simulink library "simeventstiming1"  (Simulink 6.6)
undefined symbols (not defined in the file or in its folder): des_support, gcbh
settings Model: Creator=mclune  LastModifiedBy=aapte  ExtModeAutoUpdateStatusClock=off

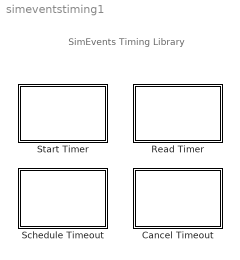
== system simeventstiming1 ==
  note: SimEvents Timing Library
  Cancel Timeout : Subsystem  Priority=0  LoadFcn=des_support('desLoadFcn',gcbh)  StartFcn=des_support('desStartFcn',gcbh)  StopFcn=des_support('desStopFcn',gcbh)  mask(Cancel Timeout){TimeoutTag=TO1, TimeoutModeOption=Continue, TimeoutCancelledOption=Error, StatNumberDeparted=Off, StatTimeoutNumberDeparted=Off, StatResidualTimeout=Off, StatAverageResidualTimeout=Off}
      mask prompts: TimeoutTag "Timeout tag:"; TimeoutModeOption "If entity does not have tagged timeout:"; TimeoutCancelledOption "If tagged timeout is not scheduled:"; StatNumberDeparted "Number of entities departed, #d:"; StatTimeoutNumberDeparted "Number of entities departed with specified tag, #t:"; StatResidualTimeout "Residual time, rt:"; StatAverageResidualTimeout "Average residual time, w:"
      mask help: Cancel specified timeout event for each tagged entity.
      mask init:
      | des_canceltimeoutmask(gcb,'init','apply');
      settings: CopyFcn=des_support('desCopyFcn',gcbh)  DeleteFcn=des_support('desDeleteFcn',gcbh)  UndoDeleteFcn=des_support('desUndoDeleteFcn',gcbh)  ModelCloseFcn=des_support('desModelCloseFcn',gcbh)  PreSaveFcn=des_support('desPreSaveFcn',gcbh)  PostSaveFcn=des_support('desPostSaveFcn',gcbh)  NameChangeFcn=des_support('desNameChangeFcn',gcbh)  CloseFcn=des_support('desCloseFcn',gcbh)  ErrorFcn=des_error_redirect
      mask Help: helpview(simeventsbhelp)
      mask StyleString: edit,popup(Error|Warn and continue|Continue),popup(Error|Warn and continue|Continue),popup(Off|On|Upon stop or pause),popup(Off|On|Upon stop or pause),popup(Off|On),popup(Off|On|Upon stop or pause)
      mask CallbackString: |||des_canceltimeoutmask(gcb,'cbStatNumberDeparted','noapply');|des_canceltimeoutmask(gcb,'cbStatTimeoutNumberDeparted','noapply');|des_canceltimeoutmask(gcb,'cbStatResidualTimeout','noapply');|des_canceltimeoutmask(gcb,'cbStatAverageResidualTimeout','noapply');
      mask TabNameString: Cancel Timeout,Cancel Timeout,Cancel Timeout,Statistics,Statistics,Statistics,Statistics
      mask Display:
      | image(des_iconLoad('timeoutCancel.jpg'),'center');
      | port_label('LConn',1,'IN');
      | port_label('RConn',1,'OUT');
  Read Timer : Subsystem  Priority=0  LoadFcn=des_support('desLoadFcn',gcbh)  StartFcn=des_support('desStartFcn',gcbh)  StopFcn=des_support('desStopFcn',gcbh)  mask(Read Timer){TimerTag=T1, TimerModeOption=Error, TimerStop=off, StatNumberDeparted=Off, StatTimerNumberDeparted=Off, StatTimeElapsed=Off, StatAverageTimeElapsed=Off}
      mask prompts: TimerTag "Timer tag:"; TimerModeOption "If entity does not have tagged timer:"; TimerStop "Stop Timer:"; StatNumberDeparted "Number of entities departed, #d:"; StatTimerNumberDeparted "Number of entities departed with specified tag, #t:"; StatTimeElapsed "Elapsed time, et:"; StatAverageTimeElapsed "Average elapsed time, w:"
      mask help: Report the instantaneous elapsed time for each tagged entity and average elapsed time for all tagged entities. The Timer tag parameter associates this block with the corresponding Start Timer block.
      mask init:
      | des_readtimermask(gcb,'init','apply');
      settings: CopyFcn=des_support('desCopyFcn',gcbh)  DeleteFcn=des_support('desDeleteFcn',gcbh)  UndoDeleteFcn=des_support('desUndoDeleteFcn',gcbh)  ModelCloseFcn=des_support('desModelCloseFcn',gcbh)  PreSaveFcn=des_support('desPreSaveFcn',gcbh)  PostSaveFcn=des_support('desPostSaveFcn',gcbh)  NameChangeFcn=des_support('desNameChangeFcn',gcbh)  CloseFcn=des_support('desCloseFcn',gcbh)  ErrorFcn=des_error_redirect
      mask Help: helpview(simeventsbhelp)
      mask StyleString: edit,popup(Error|Ignore),checkbox,popup(Off|On|Upon stop or pause),popup(Off|On|Upon stop or pause),popup(Off|On),popup(Off|On|Upon stop or pause)
      mask CallbackString: |||des_readtimermask(gcb,'cbStatNumberDeparted','noapply');|des_readtimermask(gcb,'cbStatTimerNumberDeparted','noapply');|des_readtimermask(gcb,'cbTimeElapsed','noapply');|des_readtimermask(gcb,'cbStatAverageTimeElapsed','noapply');
      mask TabNameString: Read Timer,Read Timer,Read Timer,Statistics,Statistics,Statistics,Statistics
      mask Display:
      | image(des_iconLoad('timerRead.jpg'),'center');
      | port_label('LConn',1,'IN');
      | port_label('RConn',1,'OUT');
  Schedule Timeout : Subsystem  Priority=0  LoadFcn=des_support('desLoadFcn',gcbh)  StartFcn=des_support('desStartFcn',gcbh)  StopFcn=des_support('desStopFcn',gcbh)  mask(Schedule Timeout){TimeoutTag=TO1, TimeoutIntervalFrom=Dialog, TimeoutInterval=1, AttributeName=TimeoutAttribute, PriorityTimeout=1700, TimeoutScheduledOption=Error, TimeoutNoDestination=Error, StatNumberDeparted=Off}
      mask prompts: TimeoutTag "Timeout tag:"; TimeoutIntervalFrom "Timeout interval from:"; TimeoutInterval "Timeout interval:"; AttributeName "Attribute name:"; PriorityTimeout "Timeout event priority:"; TimeoutScheduledOption "If timeout is already scheduled:"; TimeoutNoDestination "If entity has no destination when timeout occurs:"; StatNumberDeparted "Number of entities departed, #d:"
      mask help: Define the beginning of a timeout region by scheduling a timeout event for each passing entity.
      mask init:
      | des_scheduletimeoutmask(gcb,'init','apply');
      settings: CopyFcn=des_support('desCopyFcn',gcbh)  DeleteFcn=des_support('desDeleteFcn',gcbh)  UndoDeleteFcn=des_support('desUndoDeleteFcn',gcbh)  ModelCloseFcn=des_support('desModelCloseFcn',gcbh)  PreSaveFcn=des_support('desPreSaveFcn',gcbh)  PostSaveFcn=des_support('desPostSaveFcn',gcbh)  NameChangeFcn=des_support('desNameChangeFcn',gcbh)  CloseFcn=des_support('desCloseFcn',gcbh)  ErrorFcn=des_error_redirect
      mask Help: helpview(simeventsbhelp)
      mask StyleString: edit,popup(Dialog|Signal port ti|Attribute),edit,edit,edit,popup(Error|Warn and reschedule|Reschedule),popup(Error|Warn and discard the entity),popup(Off|On|Upon stop or pause)
      mask CallbackString: |des_scheduletimeoutmask(gcb,'cbTimeoutIntervalFrom','noapply');||||||
      mask TabNameString: Schedule Timeout,Schedule Timeout,Schedule Timeout,Schedule Timeout,Schedule Timeout,Schedule Timeout,Schedule Timeout,Statistics
      mask Display:
      | image(des_iconLoad('timeoutSchedule.jpg'),'center');
      | port_label('LConn',1,'IN');
      | port_label('RConn',1,'OUT');
  Start Timer : Subsystem  Priority=0  LoadFcn=des_support('desLoadFcn',gcbh)  StartFcn=des_support('desStartFcn',gcbh)  StopFcn=des_support('desStopFcn',gcbh)  mask(Start Timer){TimerTag=T1, TimerStartedOption=Warn and continue, StatNumberDeparted=Off}
      mask prompts: TimerTag "Timer tag:"; TimerStartedOption "If timer has already started:"; StatNumberDeparted "Number of entities departed, #d:"
      mask help: Define the beginning of a timer region for each entity. The Timer tag parameter associates this block with the corresponding Read Timer block.
      mask init:
      | des_starttimermask(gcb,'init','apply');
      settings: CopyFcn=des_support('desCopyFcn',gcbh)  DeleteFcn=des_support('desDeleteFcn',gcbh)  UndoDeleteFcn=des_support('desUndoDeleteFcn',gcbh)  ModelCloseFcn=des_support('desModelCloseFcn',gcbh)  PreSaveFcn=des_support('desPreSaveFcn',gcbh)  PostSaveFcn=des_support('desPostSaveFcn',gcbh)  NameChangeFcn=des_support('desNameChangeFcn',gcbh)  CloseFcn=des_support('desCloseFcn',gcbh)  ErrorFcn=des_error_redirect
      mask Help: helpview(simeventsbhelp)
      mask StyleString: edit,popup(Warn and continue|Continue|Restart),popup(Off|On|Upon stop or pause)
      mask TabNameString: Start Timer,Start Timer,Statistics
      mask Display:
      | image(des_iconLoad('timerStart.jpg'),'center');
      | port_label('LConn',1,'IN');
      | port_label('RConn',1,'OUT');

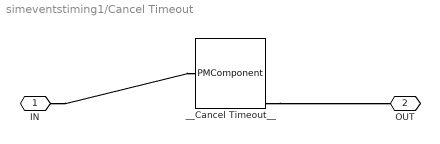
== system simeventstiming1/Cancel Timeout ==
  __Cancel Timeout__ : PMComponent  PhysicalDomain=simevents  SubClassName=DES_CANCELTIMEOUT  LeftPortType=desPortIn  RightPortType=desPortOut  IconImage=body_q.bmp  LConnTagsString=DI  RConnTagsString=DO|DO|DO|DO|DO
      mask Display:
      | port_label('LConn',1,'IN');
      | port_label('RConn',1,'#d');
      | port_label('RConn',2,'#t');
      | port_label('RConn',3,'rt');
      | port_label('RConn',4,'w');
      | port_label('RConn',5,'OUT');
  IN : PMIOPort  Port=1  Side=Left
  OUT : PMIOPort  Orientation=left  Port=2  Side=Right
  connections:
  IN/RConn1 -- __Cancel Timeout__/LConn1
  __Cancel Timeout__/RConn5 -- OUT/RConn1

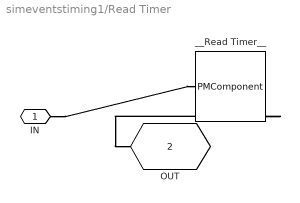
== system simeventstiming1/Read Timer ==
  __Read Timer__ : PMComponent  PhysicalDomain=simevents  SubClassName=DES_READTIMER  LeftPortType=desPortIn  RightPortType=desPortOut  IconImage=body_q.bmp  LConnTagsString=DI  RConnTagsString=DO|DO|DO|DO|DO
      mask Display:
      | port_label('LConn',1,'IN');
      | port_label('RConn',1,'#d');
      | port_label('RConn',2,'#t');
      | port_label('RConn',3,'et');
      | port_label('RConn',4,'w');
      | port_label('RConn',5,'OUT');
  IN : PMIOPort  Port=1  Side=Left
  OUT : PMIOPort  Orientation=left  Port=2  Side=Right
  connections:
  IN/RConn1 -- __Read Timer__/LConn1
  __Read Timer__/RConn5 -- OUT/RConn1

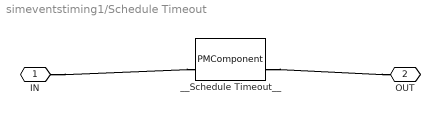
== system simeventstiming1/Schedule Timeout ==
  __Schedule Timeout__ : PMComponent  PhysicalDomain=simevents  SubClassName=DES_SCHEDULETIMEOUT  LeftPortType=desPortIn  RightPortType=desPortOut  IconImage=body_q.bmp  LConnTagsString=DI|DI  RConnTagsString=DO|DO
      mask Display:
      | port_label('LConn',1,'ti');
      | port_label('LConn',2,'IN');
      | port_label('RConn',1,'#d');
      | port_label('RConn',2,'OUT');
  IN : PMIOPort  Port=1  Side=Left
  OUT : PMIOPort  Orientation=left  Port=2  Side=Right
  connections:
  IN/RConn1 -- __Schedule Timeout__/LConn2
  __Schedule Timeout__/RConn2 -- OUT/RConn1

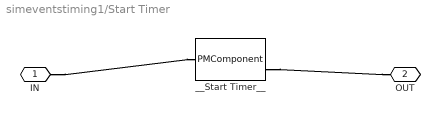
== system simeventstiming1/Start Timer ==
  __Start Timer__ : PMComponent  PhysicalDomain=simevents  SubClassName=DES_STARTTIMER  LeftPortType=desPortIn  RightPortType=desPortOut  IconImage=body_q.bmp  LConnTagsString=DI  RConnTagsString=DO|DO
      mask Display:
      | port_label('LConn',1,'IN');
      | port_label('RConn',1,'#d');
      | port_label('RConn',2,'OUT');
  IN : PMIOPort  Port=1  Side=Left
  OUT : PMIOPort  Orientation=left  Port=2  Side=Right
  connections:
  IN/RConn1 -- __Start Timer__/LConn1
  __Start Timer__/RConn2 -- OUT/RConn1
